simulink model "mucsleAcivation"  (R2017a)
settings: Solver=VariableStepAuto  StartTime=0.0  StopTime=10.0  RelTol=1e-3
settings Model: Creator=Nathaniel  LastModifiedBy=Nathaniel

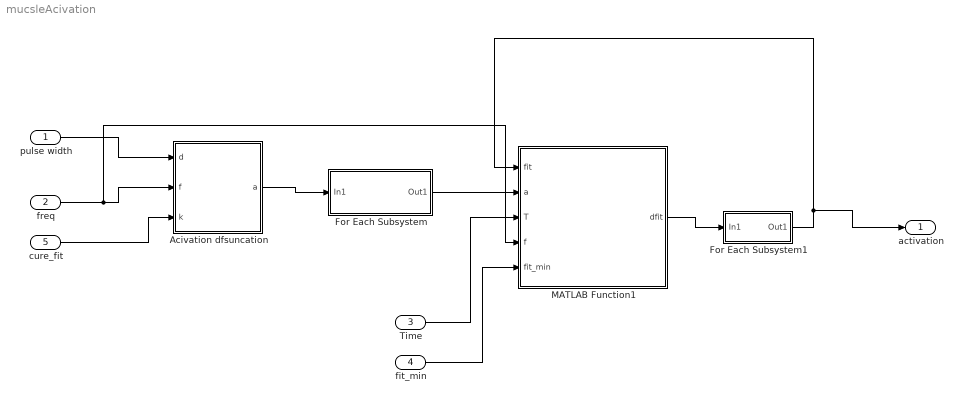
== system mucsleAcivation ==
  " pulse width " : Inport
  "freq " : Inport  Port=2
  "Time " : Inport  Port=3
  "fit_min " : Inport  Port=4
  "cure_fit " : Inport  Port=5
  Acivation dfsuncation : MATLAB Function  TreatAsAtomicUnit=on
  For Each Subsystem : Subsystem  TreatAsAtomicUnit=on
  For Each Subsystem1 : Subsystem  TreatAsAtomicUnit=on
  MATLAB Function1 : MATLAB Function  TreatAsAtomicUnit=on
  "activation " : Outport
  wires:
  Acivation dfsuncation/1(a) -> For Each Subsystem/1(In1)
  For Each Subsystem/1(Out1) -> MATLAB Function1/2(a)
  " pulse width "/1 -> Acivation dfsuncation/1(d)
  "freq "/1 -> MATLAB Function1/4(f), Acivation dfsuncation/2(f)
  "Time "/1 -> MATLAB Function1/3(T)
  "fit_min "/1 -> MATLAB Function1/5(fit_min)
  For Each Subsystem1/1(Out1) -> "activation "/1, MATLAB Function1/1(fit)
  "cure_fit "/1 -> Acivation dfsuncation/3(k)
  MATLAB Function1/1(dfit) -> For Each Subsystem1/1(In1)

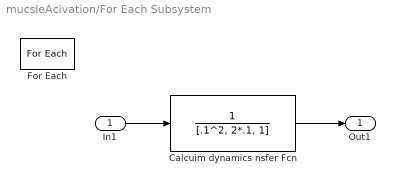
== system mucsleAcivation/For Each Subsystem ==
  In1 : Inport  Partition=on  PartitionDimension=1  PartitionWidth=1
  Calcuim dynamics nsfer Fcn : TransferFcn  Denominator=[.1^2, 2*.1, 1]
  For Each : ForEach  DisableCoverage=on  IndexMode=One-based
  Out1 : Outport  ConcatenationDimension=1
  wires:
  In1/1 -> Calcuim dynamics nsfer Fcn/1
  Calcuim dynamics nsfer Fcn/1 -> Out1/1

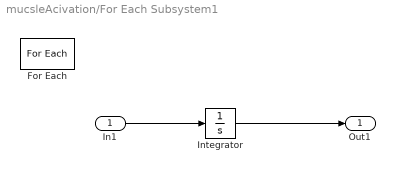
== system mucsleAcivation/For Each Subsystem1 ==
  In1 : Inport  Partition=on  PartitionDimension=1  PartitionWidth=1
  For Each : ForEach  DisableCoverage=on  IndexMode=One-based
  Integrator : Integrator
  Out1 : Outport  ConcatenationDimension=1
  wires:
  In1/1 -> Integrator/1
  Integrator/1 -> Out1/1

== matlab function mucsleAcivation/MATLAB Function1 ==
  data: fit input; a input; T input; dfit output; f input; fit_min input
function dfit = fcn( fit,a,T,f,fit_min )

dfit = fatigue( fit,a,T,f,fit_min );

== matlab function mucsleAcivation/Acivation dfsuncation ==
  data: d input; a output; f input; k input
function a = fcn(d,f,k)

a = activation(d,f,k);
